simulink model "retro_positiva_sim"  (Simulink 7.1)
settings: Solver=ode5  StartTime=0.0  StopTime=500  FixedStep=0.001  RelTol=1e-3
settings Model: Creator=Usuario  LastModifiedBy=Usuario  ExtModeTrigDuration=10000
settings SolverCC: PositivePriorityOrder=on
settings OptimizationCC: ExpressionDepthLimit=128  InitFltsAndDblsToZero=off
settings DebuggingCC: SolverPrmCheckMsg=none  FcnCallInpInsideContextMsg=Enable All  StateNameClashWarn=none  StrictBusMsg=ErrorLevel1
settings RTWCC: SystemTargetFile=quarc_win64.tlc  TemplateMakefile=quarc_default_tmf  Description=QUARC Win64 Target
settings CodeAppCC: CustomSymbolStrType=$N$R$M_T
settings STFCustomTargetCC: TargetPreCompLibLocation=C:\PROGRA~3\QUARC\lib\2015a\win64\release  TargetFunctionLibrary=C89/C90 (ANSI)  ConcurrentExecutionCompliant=on  MatFileLogging=on  SystemTargetFile=quarc_win64.tlc
settings GRTTargetCC: TargetPreCompLibLocation=C:\PROGRA~3\QUARC\lib\2015a\win64\release  TargetFunctionLibrary=C89/C90 (ANSI)  CompOptLevelCompliant=off  CPPClassGenCompliant=off  ExtMode=on  ExtModeMexFile=quarc_comm

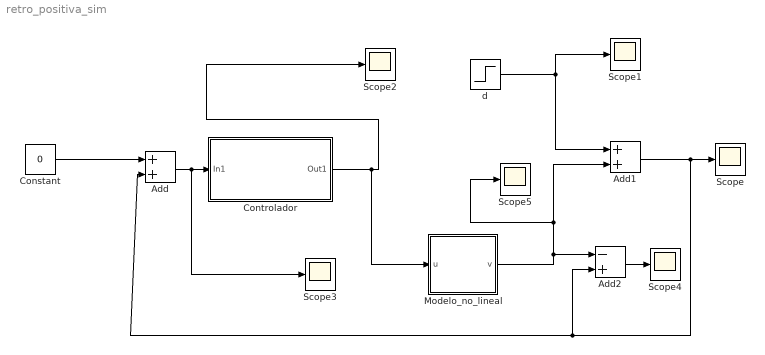
== system retro_positiva_sim ==
  Add : Sum
  Add1 : Sum
  Add2 : Sum  Inputs=-+
  Constant : Constant  Value=0
  Controlador : Subsystem
  Modelo_no_lineal : Subsystem
  Scope{,1..5} (6 alike) : Scope
      Scope settings: TimeRange=50  YMin=-15  YMax=20
      Scope2 settings: SaveName=ScopeData2
      Scope3 settings: YMin=20  YMax=20  SaveName=ScopeData3
      Scope4 settings: TimeRange=50  YMin=-15  YMax=20  SaveName=ScopeData4
      Scope5 settings: SaveName=ScopeData5
  d : Step  Time=0  SampleTime=0
  wires:
  Constant/1 -> Add/1
  Add/1 -> Scope3/1, Controlador/1(In1)
  Add1/1 -> Add2/2, Add/2, Scope/1
  d/1 -> Scope1/1, Add1/1
  Controlador/1(Out1) -> Modelo_no_lineal/1(u), Scope2/1
  Modelo_no_lineal/1(v) -> Add2/1, Add1/2, Scope5/1
  Add2/1 -> Scope4/1

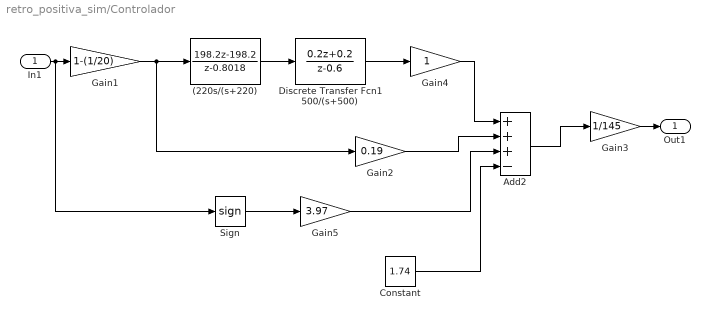
== system retro_positiva_sim/Controlador ==
  In1 : Inport
  (220s/(s+220) : DiscreteTransferFcn  Numerator=[198.2 -198.2]  Denominator=[1 -0.8018]  SampleTime=0.001
  Add2 : Sum  Inputs=+++-
  Constant : Constant  Value=1.74
  Discrete Transfer Fcn1 500/(s+500) : DiscreteTransferFcn  Numerator=[0.2 0.2]  Denominator=[1 -0.6]  SampleTime=0.001
  Gain1 : Gain  Gain=1-(1/20)
  Gain2 : Gain  Gain=0.19
  Gain3 : Gain  Gain=1/145
  Gain4 : Gain
  Gain5 : Gain  Gain=3.97
  Sign : Signum
  Out1 : Outport
  wires:
  Gain1/1 -> (220s/(s+220)/1, Gain2/1
  Gain3/1 -> Out1/1
  Gain2/1 -> Add2/2
  Add2/1 -> Gain3/1
  (220s/(s+220)/1 -> Discrete Transfer Fcn1 500/(s+500)/1
  Discrete Transfer Fcn1 500/(s+500)/1 -> Gain4/1
  Gain4/1 -> Add2/1
  In1/1 -> Sign/1, Gain1/1
  Sign/1 -> Gain5/1
  Gain5/1 -> Add2/3
  Constant/1 -> Add2/4

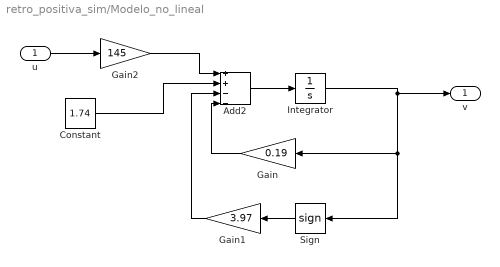
== system retro_positiva_sim/Modelo_no_lineal ==
  u : Inport
  Add2 : Sum  Inputs=++--
  Constant : Constant  Value=1.74
  Gain : Gain  Orientation=left  Gain=0.19
  Gain1 : Gain  Orientation=left  Gain=3.97
  Gain2 : Gain  Gain=145
  Integrator : Integrator  InitialCondition=0.1
  Sign : Signum  Orientation=left
  v : Outport
  wires:
  Sign/1 -> Gain1/1
  u/1 -> Gain2/1
  Integrator/1 -> v/1, Sign/1, Gain/1
  Gain2/1 -> Add2/1
  Add2/1 -> Integrator/1
  Gain/1 -> Add2/4
  Gain1/1 -> Add2/3
  Constant/1 -> Add2/2
